simulink model "transfer_fun1"  (R2016a)
settings: Solver=VariableStepAuto  StartTime=0.0  StopTime=10.0  RelTol=1e-3
undefined symbols (not defined in the file or in its folder): E, L, R
settings Model: Creator=Ronok  LastModifiedBy=Ronok

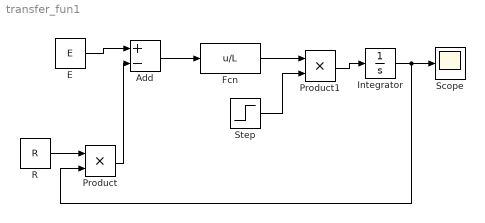
== system transfer_fun1 ==
  Add : Sum  Inputs=+-
  E : Constant  Value=E
  Fcn : Fcn  Expr=u/L
  Integrator : Integrator
  Product : Product
  Product1 : Product
  R : Constant  Value=R
  Scope : Scope
  Step : Step  Time=.5  SampleTime=0
  wires:
  E/1 -> Add/1
  R/1 -> Product/1
  Product/1 -> Add/2
  Integrator/1 -> Scope/1, Product/2
  Add/1 -> Fcn/1
  Fcn/1 -> Product1/1
  Step/1 -> Product1/2
  Product1/1 -> Integrator/1
